simulink model "Feedback_Petko_Modeling_Different"  (R2015a)
settings: Solver=ode5  StartTime=0.0  StopTime=20  FixedStep=0.001  MaxStep=0.01  RelTol=1e-3
undefined symbols (not defined in the file): sigbuilder_block
settings Model: Creator=Fares  LastModifiedBy=Fares

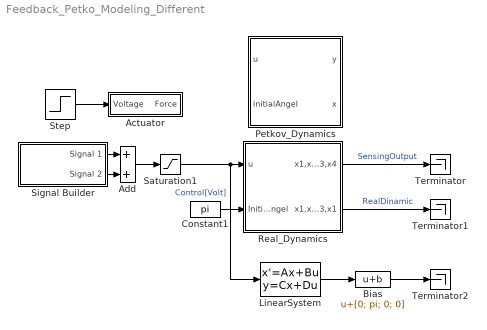
== system Feedback_Petko_Modeling_Different ==
  Actuator : Subsystem
  Add : Sum
  Bias : Bias  Bias=[0; pi; 0; 0]
  Constant1 : Constant  Value=pi
  LinearSystem : StateSpace  A=A  B=B  C=C  D=D  X0=[0; 0; 0; 0]  mask(SS MASK){}
      mask init:
      | mc = 1.12;
      | mpw = 0.095;
      | mps = 0.025;
      | l = 0.0167903; % lco = 0.347;
      | fc = 2.53165; % FS = 2.53165; FC = 2.28133
      | fp = 0.000107443;
      | J = 0.0135735;
      | g = 9.81;
      | vf = 17.463/2.5; %Voltage to Motor Force ratio
      | mp = mpw + mps;
      | a = l^2 + J/(mc + mp);
      | mu = (mc + mp)*l;
      | 
      | % theta 0 in upward position
      | % theta pi in downward position
      | s = -1; % 1 when upward  -1 when downward
      | 
      | A = [0          0              1               0;
      |      0          0              0               1;
      |      0      (l*mu*g)/J    -(a*fc)/J    -(l*fp)/J;
      |      0      s*(mu*g)/J    -s*(l*fc)/J    -(fp)/J];
      |  
      | B = [         0;
      |               0;
      |        (vf*a)/J;
      |       (s*vf*l)/J];
      |   
      | C = [1 0 0 0;
      |      0 1 0 0;
      |      0 0 1 0;
      |      0 0 0 1];
      |  
      | D = [0;
      |      0;
      |      0;
      |      0];
  Petkov_Dynamics : Subsystem  mask{mp=0.95 + 0.025, mc=1.12, l=0.347, I=0.0135735, fc=2.53165, fp=0.000107443, kf=17.463, g=-9.81}
      mask prompts: mp "Pedulum mass [kg]"; mc "Cart mass [kg]"; l "Distance from the base to the system CoM [m]"; I "Pendulum of moment of inertia [kg*m2]"; fc "Dynamic cart friction [N s/m]"; fp "Rotational friction [N ms/rad]"; kf "Control  force to PWM signal ratio [N]"; g "Gravitational acceleration [m/s2]"
      mask init:
      | Mt = mc + mp;
      | It = I + mp*l^2;
  Real_Dynamics : Subsystem  mask{mc=1.12, mpw=0.095, mps=0.025, M=17.463, fp=0.000107443, J=0.0135735, l=0.0167903, g=9.81}
      mask prompts: mc "Cart mass [kg]"; mpw "Pendulum weight mass [kg]"; mps "Pendulum stick mass [kg]"; M "Maximum control [N]"; fp "Pendulum friction [kg*m2/s]"; J "Moment of inertia [kg*m2]"; l "Distance: axis of rotation-mass center [m]"; g "Gravetational acceleration [m/s2]"
      mask init:
      | mp = mpw + mps;
      | a = l^2 + J/(mc + mp);
      | mi = (mc + mp)*l;
      mask Display: plot([0 0],[-2.5 4.5],[5 5],[-2.5 4.5],[0 5],[0 0],[0 5],[0.1 0.1],[0 2],[1 1],[2.5 5],[1 1],[2 2.5 2.5 2 2],[1.25 1.25 0.75 0.75 1.25],[2.25 1.5],[1 -2.5]);
  Saturation1 : Saturate  UpperLimit=2.5  LowerLimit=-2.5
  Signal Builder : Subsystem  Tag=STV Subsys  LoadFcn=sigbuilder_block('load');  StartFcn=sigbuilder_block('start');  StopFcn=sigbuilder_block('stop');  ClipboardFcn=sigbuilder_block('clipboard');  mask(Sigbuilder block){}
      mask help: Simulink:masks:SigbuilderBlock_MD
      mask init:
      | if ~strcmp(get_param(bdroot(gcbh),'SimulationStatus'),'stopped') tuvar = sigbuilder_block('maskInit'); end
      settings: CopyFcn=sigbuilder_block('copy');  DeleteFcn=sigbuilder_block('delete');  ModelCloseFcn=sigbuilder_block('modelClose');  PreSaveFcn=sigbuilder_block('preSave');  PauseFcn=sigbuilder_block('pause');  ContinueFcn=sigbuilder_block('continue');  NameChangeFcn=sigbuilder_block('namechange');  OpenFcn=sigbuilder_block('open',[437.6 199.2 550.4 400 ]);  CloseFcn=sigbuilder_block('close');
      mask Display: plot(0, 0, 100, 100,[2, 2, 32, 32, 2], [68, 8, 8, 68, 68],[32, 2], [38, 38], [32, 19, 2],[53, 60, 44], [32, 17, 17, 2],[16, 16, 31, 31]);txt = getActiveGroup(gcbh);text(2, 100, txt,'verticalAlignment', 'top');
  Step : Step  Time=0.2  Before=24  After=0  SampleTime=0
  Terminator : Terminator
  Terminator1 : Terminator
  Terminator2 : Terminator
  wires:
  Step/1 -> Actuator/1(Voltage)
  Constant1/1 -> Real_Dynamics/2(Initial_Angel)
  Add/1 -> Saturation1/1
  Signal Builder/1(Signal 1) -> Add/1
  Saturation1/1 -> LinearSystem/1, Real_Dynamics/1(u)  "Control[Volt]"
  Real_Dynamics/1(x1,x2,x3,x4) -> Terminator/1  "SensingOutput"
  Real_Dynamics/2(x1,x2,x3,x1) -> Terminator1/1  "RealDinamic"
  Signal Builder/2(Signal 2) -> Add/2
  LinearSystem/1 -> Bias/1
  Bias/1 -> Terminator2/1

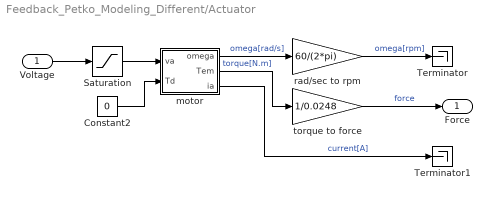
== system Feedback_Petko_Modeling_Different/Actuator ==
  Voltage : Inport
  Constant2 : Constant  Value=0
  Saturation : Saturate  UpperLimit=25  LowerLimit=-25
  Terminator : Terminator
  Terminator1 : Terminator
  motor : Subsystem  mask{J=140e-7, b=3.6092e-5, Ke=0.052, Kt=0.052, Ra=2.5, La=2.5e-3}
      mask prompts: J "Moment of inertia of the rotor [Kg.m2]"; b "Motor viscous friction constant [N.m.s]"; Ke "Electromotive force constant [V/rad/sec]"; Kt "Motor torque constant [N.m/Amp]"; Ra "Electric resistance [ohm]"; La "Electric inductance [H]"
  rad/sec to rpm : Gain  Gain=60/(2*pi)
  torque to force : Gain  Gain=1/0.0248
  Force : Outport
  wires:
  rad/sec to rpm/1 -> Terminator/1  "omega[rpm]"
  Constant2/1 -> motor/2(Td)
  Voltage/1 -> Saturation/1
  motor/1(omega) -> rad/sec to rpm/1  "omega[rad/s]"
  Saturation/1 -> motor/1(va)
  motor/2(Tem) -> torque to force/1  "torque[N.m]"
  torque to force/1 -> Force/1  "force"
  motor/3(ia) -> Terminator1/1  "current[A]"

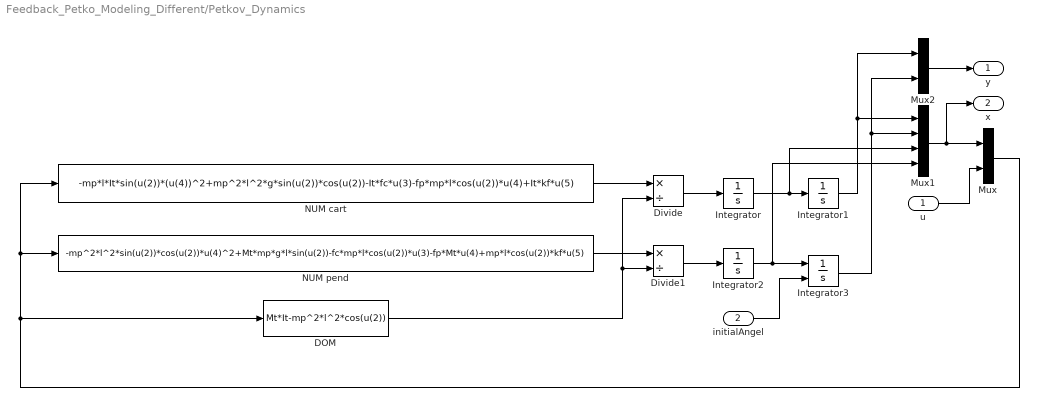
== system Feedback_Petko_Modeling_Different/Petkov_Dynamics ==
  u : Inport
  initialAngel : Inport  Port=2
  "DOM " : Fcn  Expr=Mt*It-mp^2*l^2*cos(u(2))
  Divide : Product  Inputs=*/
  Divide1 : Product  Inputs=*/
  Integrator : Integrator
  Integrator1 : Integrator
  Integrator2 : Integrator
  Integrator3 : Integrator  InitialConditionSource=external  InitialCondition=pi
  Mux : Mux  Inputs=2
  Mux1 : Mux
  Mux2 : Mux  Inputs=2
  "NUM cart " : Fcn  Expr=-mp*l*It*sin(u(2))*(u(4))^2+mp^2*l^2*g*sin(u(2))*cos(u(2))-It*fc*u(3)-fp*mp*l*cos(u(2))*u(4)+It*kf*u(5)
  NUM pend : Fcn  Expr=-mp^2*l^2*sin(u(2))*cos(u(2))*u(4)^2+Mt*mp*g*l*sin(u(2))-fc*mp*l*cos(u(2))*u(3)-fp*Mt*u(4)+mp*l*cos(u(2))*kf*u(5)
  y : Outport
  x : Outport  Port=2
  wires:
  "NUM cart "/1 -> Divide/1
  NUM pend/1 -> Divide1/1
  "DOM "/1 -> Divide/2, Divide1/2
  Mux/1 -> "NUM cart "/1, NUM pend/1, "DOM "/1
  Divide/1 -> Integrator/1
  Integrator2/1 -> Mux1/4, Integrator3/1
  u/1 -> Mux/2
  Divide1/1 -> Integrator2/1
  Integrator1/1 -> Mux2/1, Mux1/1
  Integrator3/1 -> Mux2/2, Mux1/2
  initialAngel/1 -> Integrator3/2
  Integrator/1 -> Mux1/3, Integrator1/1
  Mux1/1 -> x/1, Mux/1
  Mux2/1 -> y/1

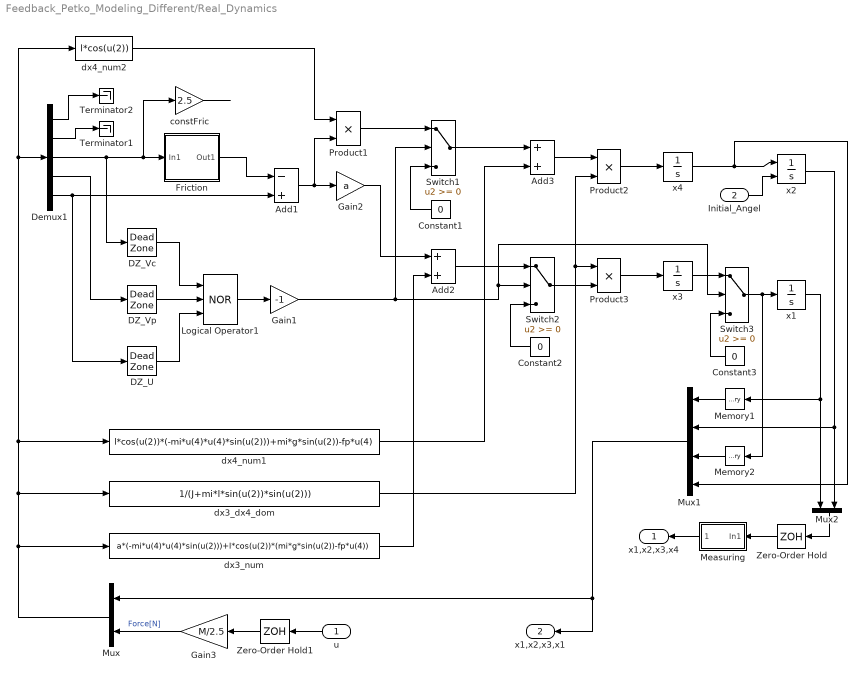
== system Feedback_Petko_Modeling_Different/Real_Dynamics ==
  u : Inport
  Initial_Angel : Inport  Port=2
  " DZ_Vp" : DeadZone  LowerValue=-3.37476  UpperValue=3.37476  SaturateOnIntegerOverflow=on
  Add1 : Sum  Inputs=-+
  Add2 : Sum
  Add3 : Sum
  Constant1 : Constant  Value=0
  Constant2 : Constant  Value=0
  Constant3 : Constant  Value=0
  DZ_U : DeadZone  LowerValue=-1.37918  UpperValue=1.37918  SaturateOnIntegerOverflow=on
  DZ_Vc : DeadZone  LowerValue=-0.00793711  UpperValue=0.00793711  SaturateOnIntegerOverflow=on
  Demux1 : Demux  Outputs=5
  Friction : Subsystem  mask{FS=2.53165, FC=2.28133, DZcv=0.00793711, Xc=0.5, Yc=2.3}
      mask prompts: FS "Static friction [N]"; FC "Coulombic friction [N]"; DZcv "Minimum cart velocity [rad/s]"; Xc "Cart velocity - beginning of the linear dependence zone [m/s]"; Yc "Friction value for Xc point [N]"
      mask init:
      | small = DZcv;
      mask Display: plot([-4 4],[0 0],[-3.8 -2.4 -1.8 -1.2 -0.6 -0.2 0 0.2 0.6 1.2 1.8 2.4 3.8],[-1.4 -1 -1.1 -1.3 -1.6 -2 0 2 1.6 1.3 1.1 1 1.4]);
  Gain1 : Gain  Gain=-1
  Gain2 : Gain  Gain=a
  Gain3 : Gain  Gain=M/2.5
  Logical Operator1 : Logic  Operator=NOR  Inputs=3  AllPortsSameDT=off  OutDataTypeStr=boolean
  Measuring : Subsystem
  Memory1 : Memory
  Memory2 : Memory
  Mux : Mux  Inputs=2
  Mux1 : Mux
  Mux2 : Mux  Inputs=2
  Product1 : Product
  Product2 : Product
  Product3 : Product
  Switch1 : Switch
  Switch2 : Switch
  Switch3 : Switch
  Terminator1 : Terminator
  Terminator2 : Terminator
  Zero-Order Hold : ZeroOrderHold  SampleTime=0.001
  Zero-Order Hold1 : ZeroOrderHold  SampleTime=0.001
  constFric : Gain  Gain=2.5
  dx3_dx4_dom : Fcn  Expr=1/(J+mi*l*sin(u(2))*sin(u(2)))
  dx3_num : Fcn  Expr=a*(-mi*u(4)*u(4)*sin(u(2)))+l*cos(u(2))*(mi*g*sin(u(2))-fp*u(4))
  dx4_num1 : Fcn  Expr=l*cos(u(2))*(-mi*u(4)*u(4)*sin(u(2)))+mi*g*sin(u(2))-fp*u(4)
  dx4_num2 : Fcn  Expr=l*cos(u(2))
  x1 : Integrator
  x2 : Integrator  InitialConditionSource=external  InitialCondition=pi/2
  x3 : Integrator
  x4 : Integrator
  x1,x2,x3,x4 : Outport
  x1,x2,x3,x1 : Outport  Port=2
  wires:
  DZ_U/1 -> Logical Operator1/3
  DZ_Vc/1 -> Logical Operator1/1
  Product1/1 -> Switch1/1
  Gain2/1 -> Add2/1
  Constant1/1 -> Switch1/3
  Switch2/1 -> Product3/2
  Product3/1 -> x3/1
  Logical Operator1/1 -> Gain1/1
  Constant3/1 -> Switch3/3
  Add3/1 -> Product2/1
  Demux1/1 -> Terminator2/1
  Mux/1 -> dx3_dx4_dom/1, dx4_num2/1, Demux1/1, dx4_num1/1, dx3_num/1
  dx4_num1/1 -> Add3/2
  x3/1 -> Switch3/1
  Switch3/1 -> Memory2/1, x1/1
  Add1/1 -> Gain2/1, Product1/2
  Add2/1 -> Switch2/1
  dx4_num2/1 -> Product1/1
  Demux1/3 -> constFric/1, Friction/1(In1), DZ_Vc/1
  Demux1/2 -> Terminator1/1
  Demux1/4 -> " DZ_Vp"/1
  Demux1/5 -> Add1/2, DZ_U/1
  " DZ_Vp"/1 -> Logical Operator1/2
  Switch1/1 -> Add3/1
  dx3_num/1 -> Add2/2
  Constant2/1 -> Switch2/3
  dx3_dx4_dom/1 -> Product2/2, Product3/1
  Product2/1 -> x4/1
  x4/1 -> x2/1, Mux1/4
  Memory2/1 -> Mux1/3
  Memory1/1 -> Mux1/1
  Mux1/1 -> x1,x2,x3,x1/1, Mux/1
  u/1 -> Zero-Order Hold1/1
  Friction/1(Out1) -> Add1/1
  Initial_Angel/1 -> x2/2
  Gain1/1 -> Switch1/2, Switch3/2, Switch2/2
  x2/1 -> Mux2/2, Mux1/2
  x1/1 -> Mux2/1, Memory1/1
  Measuring/1(Out1) -> x1,x2,x3,x4/1
  Mux2/1 -> Zero-Order Hold/1
  Zero-Order Hold/1 -> Measuring/1(In1)
  Zero-Order Hold1/1 -> Gain3/1
  Gain3/1 -> Mux/2  "Force[N]"
  constFric/1 -> ?

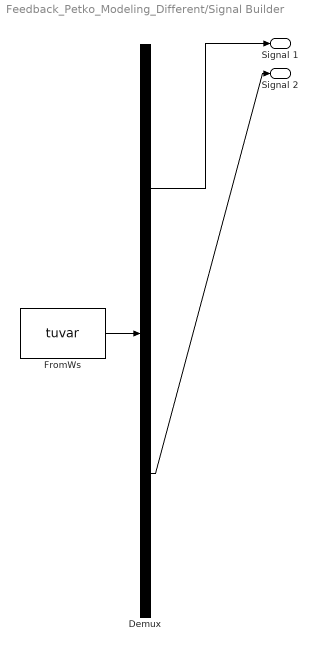
== system Feedback_Petko_Modeling_Different/Signal Builder ==
  Demux : Demux  Tag=STV Demux  Outputs=2
  FromWs : FromWorkspace  Tag=STV FromWs  VariableName=tuvar  SampleTime=0
      SigBuilderData=|
      | common.afterFinalStr = 'Extrapolate'
      | common.sampleTime = 0
      | dataSet.timeRange = [0 10]
      | dataSet.name = 'Group 1'
      | sbobj.Groups.Name = 'Group 1'
      | sbobj.Groups.Signals(1).Name = 'Signal 1'
      | sbobj.Groups.Signals(1).XData = [0 0.2 0.2 10]
      | sbobj.Groups.Signals(1).YData = [1.8 1.8 0 0]
      | sbobj.Groups.Signals(2).Name = 'Signal 2'
      | sbobj.Groups.Signals(2).XData = [0 9 9 9.2 9.2 10]
      | sbobj.Groups.Signals(2).YData = [0 0 -1.8 -1.8 0 0]
  Signal 1 : Outport  Tag=STV Outport
  Signal 2 : Outport  Tag=STV Outport  Port=2
  wires:
  Demux/1 -> Signal 1/1
  FromWs/1 -> Demux/1
  Demux/2 -> Signal 2/1

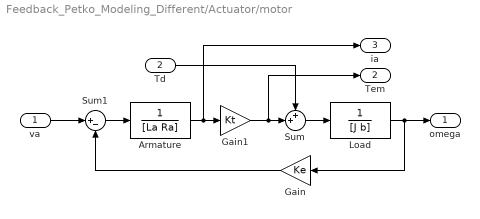
== system Feedback_Petko_Modeling_Different/Actuator/motor ==
  va : Inport
  Td : Inport  Port=2
  Armature : TransferFcn  Denominator=[La Ra]
  Gain : Gain  Gain=Ke
  Gain1 : Gain  Gain=Kt
  Load : TransferFcn  Denominator=[J b]
  Sum : Sum  Inputs=++|
  Sum1 : Sum  Inputs=|+-
  omega : Outport
  Tem : Outport  Port=2
  ia : Outport  Port=3
  wires:
  Sum/1 -> Load/1
  va/1 -> Sum1/1
  Gain/1 -> Sum1/2
  Sum1/1 -> Armature/1
  Td/1 -> Sum/1
  Gain1/1 -> Tem/1, Sum/2
  Armature/1 -> ia/1, Gain1/1
  Load/1 -> omega/1, Gain/1

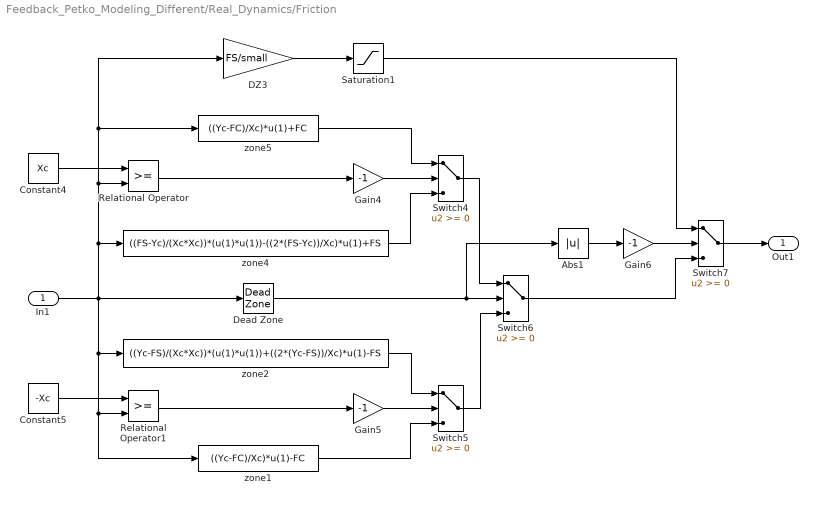
== system Feedback_Petko_Modeling_Different/Real_Dynamics/Friction ==
  In1 : Inport
  Abs1 : Abs
  Constant4 : Constant  Value=Xc
  Constant5 : Constant  Value=-Xc
  DZ3 : Gain  Gain=FS/small
  Dead Zone : DeadZone  LowerValue=-DZcv  UpperValue=DZcv  SaturateOnIntegerOverflow=on
  Gain4 : Gain  Gain=-1
  Gain5 : Gain  Gain=-1
  Gain6 : Gain  Gain=-1
  Relational Operator : RelationalOperator  OutDataTypeStr=boolean
  Relational Operator1 : RelationalOperator  OutDataTypeStr=boolean
  Saturation1 : Saturate  UpperLimit=FS  LowerLimit=-FS
  Switch{4..7} (4 alike) : Switch
  zone1 : Fcn  Expr=((Yc-FC)/Xc)*u(1)-FC
  zone2 : Fcn  Expr=((Yc-FS)/(Xc*Xc))*(u(1)*u(1))+((2*(Yc-FS))/Xc)*u(1)-FS
  zone4 : Fcn  Expr=((FS-Yc)/(Xc*Xc))*(u(1)*u(1))-((2*(FS-Yc))/Xc)*u(1)+FS
  zone5 : Fcn  Expr=((Yc-FC)/Xc)*u(1)+FC
  Out1 : Outport
  wires:
  Gain4/1 -> Switch4/2
  Dead Zone/1 -> Abs1/1, Switch6/2
  Gain5/1 -> Switch5/2
  Relational Operator/1 -> Gain4/1
  Constant5/1 -> Relational Operator1/1
  Relational Operator1/1 -> Gain5/1
  Abs1/1 -> Gain6/1
  DZ3/1 -> Saturation1/1
  Switch6/1 -> Switch7/3
  Switch4/1 -> Switch6/1
  zone2/1 -> Switch5/1
  Gain6/1 -> Switch7/2
  zone4/1 -> Switch4/3
  Switch7/1 -> Out1/1
  In1/1 -> zone1/1, Relational Operator1/2, zone2/1, DZ3/1, zone5/1, Relational Operator/2, zone4/1, Dead Zone/1
  Saturation1/1 -> Switch7/1
  zone5/1 -> Switch4/1
  Constant4/1 -> Relational Operator/1
  zone1/1 -> Switch5/3
  Switch5/1 -> Switch6/3

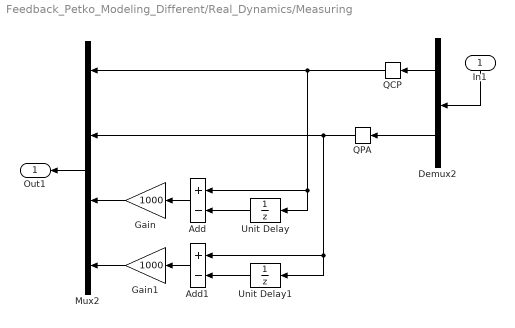
== system Feedback_Petko_Modeling_Different/Real_Dynamics/Measuring ==
  In1 : Inport
  Add : Sum  Inputs=+-
  Add1 : Sum  Inputs=+-
  Demux2 : Demux  Outputs=2
  Gain : Gain  Gain=1000
  Gain1 : Gain  Gain=1000
  Mux2 : Mux
  QCP : Quantizer  QuantizationInterval=0.156/2048
  QPA : Quantizer  QuantizationInterval=(2*pi)/2048
  Unit Delay : UnitDelay  SampleTime=-1
  Unit Delay1 : UnitDelay  SampleTime=-1
  Out1 : Outport
  wires:
  Demux2/1 -> QCP/1
  Mux2/1 -> Out1/1
  In1/1 -> Demux2/1
  QPA/1 -> Unit Delay1/1, Add1/1, Mux2/2
  QCP/1 -> Unit Delay/1, Add/1, Mux2/1
  Demux2/2 -> QPA/1
  Unit Delay1/1 -> Add1/2
  Unit Delay/1 -> Add/2
  Add1/1 -> Gain1/1
  Add/1 -> Gain/1
  Gain1/1 -> Mux2/4
  Gain/1 -> Mux2/3
